simulink model "flight_sim"  (R2024a)
settings: Solver=VariableStepAuto  StartTime=0.0  StopTime=100  RelTol=1e-3
libraries: aerolibatmos2 x1, matrix_library x1, shared6dof x1
settings Model: Creator=zach  LastModifiedBy=zach

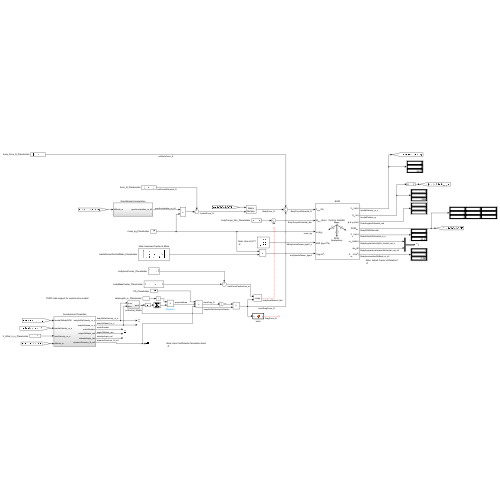
[thumbnail: Simulink's stored preview of the top-level diagram]
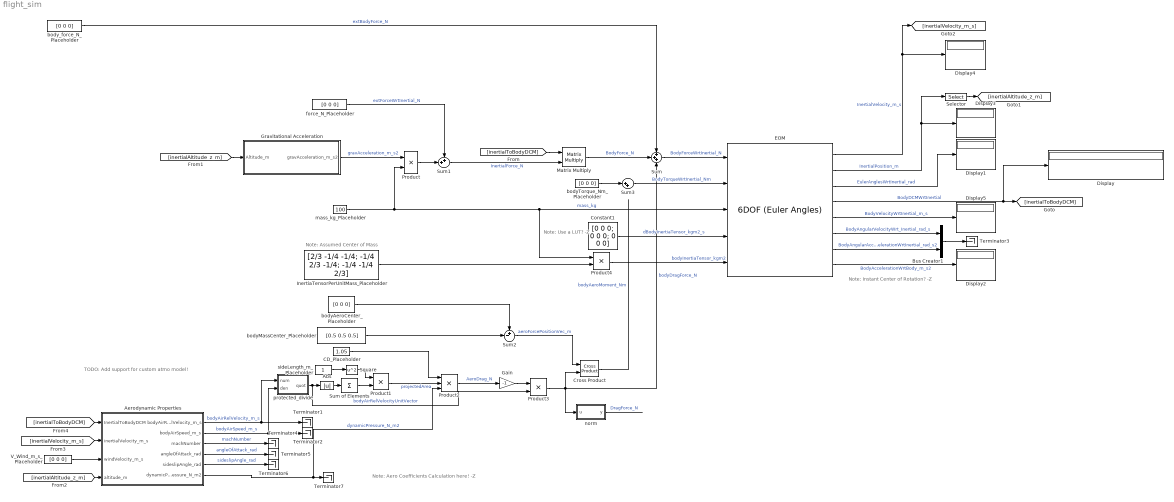
== system flight_sim ==
  note: Note: Assumed Center of Mass
  note: TODO: Add support for custom atmo model!
  note: Note: Aero Coefficients Calculation here!
      |  -Z
  note: Note: Instant Center of Rotation?
      | -Z
  note: Note: Use a LUT?
      | -Z
  Abs : Abs  SaturateOnIntegerOverflow=off
  Aerodynamic Properties : Subsystem
  Bus Creator1 : BusCreator  Inputs=2
  CD_Placeholder : Constant  Value=1.05
  Constant1 : Constant  Value=[0 0 0; 0 0 0; 0 0 0]
  Cross Product : matrix_library/Cross Product
  Display{,1..5} (6 alike) : Display
  EOM : shared6dof/6DOF (Euler Angles)  units=Metric (MKS)  mtype=Custom Variable  rep=Quaternion  xme_0=[0 0 10000]  Vm_0=[0 0 0]  eul_0=[0 0 0]  pm_0=[0 0 0]  mass_0=100  mass_e=0.5  mass_f=100  inertia=eye(3)  inertia_e=eye(3)  inertia_f=2*eye(3)  k_quat=1.0  vre_flag=off  abi_flag=off  aMode=0  xme_statename=''  Vm_statename=''  eul_statename=''  quat_statename=''  pm_statename=''  mass_statename=''
      settings: LibrarySourceBlock=aerolib6dof2/6DOF (Quaternion)
  Gain : Gain  Gain=-1
  Gravitational Acceleration : Subsystem
  InertiaTensorPerUnitMass_Placeholder : Constant  Value=[2/3 -1/4 -1/4; -1/4 2/3 -1/4; -1/4 -1/4 2/3]
  Matrix Multiply : Product  Multiplication=Matrix(*)
  Product{,1,3..4} (4 alike) : Product
  Product2 : Product  Inputs=3
  Selector : Selector  InputPortWidth=3  IndexOptions=Index vector (dialog)  Indices=[3]  OutputSizes=1
  Square : Math  Operator=square
  Sum : Sum  Inputs=+++
  Sum of Elements : Sum  Inputs=+
  Sum1 : Sum  Inputs=++|
  Sum2 : Sum  Inputs=+-|
  Sum3 : Sum  Inputs=|++
  Terminator{1..7} (7 alike) : Terminator
  V_Wind_m_s_Placeholder : Constant  Value=[0 0 0]
  bodyAeroCenter_Placeholder : Constant  Value=[0 0 0]
  bodyMassCenter_Placeholder : Constant  Value=[0.5 0.5 0.5]
  bodyTorque_Nm_Placeholder : Constant  Value=[0 0 0]
  body_force_N_Placeholder : Constant  Value=[0 0 0]
  force_N_Placeholder : Constant  Value=[0 0 0]
  mass_kg_Placeholder : Constant  Value=100
  norm : MATLAB Function  TreatAsAtomicUnit=on
  protected_divide : Subsystem
  sideLength_m_Placeholder : Constant
  wires:
  Sum3/1 -> EOM/2  "BodyTorqueWrtInertial_Nm"
  EOM/3 -> Display1/1  "EulerAnglesWrtInertial_rad"
  EOM/2 -> Selector/1, Display3/1  "InertialPosition_m"
  EOM/1 -> [inertialVelocity_m_s], Display4/1  "InertialVelocity_m_s"
  EOM/4 -> Display/1, [inertialToBodyDCM]  "BodyDCMWrtInertial"
  EOM/5 -> Display5/1  "BodyVelocityWrtInertial_m_s"
  mass_kg_Placeholder/1 -> Product4/1, EOM/3, Product/2  "mass_kg"
  Sum/1 -> EOM/1  "BodyForceWrtInertial_N"
  Constant1/1 -> EOM/4  "dBodyInertiaTensor_kgm2_s"
  Product4/1 -> EOM/5  "bodyInertiaTensor_kgm2"
  Product/1 -> Sum1/2
  EOM/6 -> Bus Creator1/1  "BodyAngularVelocityWrt_Inertial_rad_s"
  EOM/7 -> Bus Creator1/2  "BodyAngularAccelerationWrtInertial_rad_s2"
  Bus Creator1/1 -> Terminator3/1
  EOM/8 -> Display2/1  "BodyAccelerationWrtBody_m_s2"
  body_force_N_Placeholder/1 -> Sum/1  "extBodyForce_N"
  force_N_Placeholder/1 -> Sum1/1  "extForceWrtInertial_N"
  Sum1/1 -> Matrix Multiply/2  "InertialForce_N"
  [inertialToBodyDCM] -> Matrix Multiply/1
  Matrix Multiply/1 -> Sum/2  "BodyForce_N"
  Selector/1 -> [inertialAltitude_z_m]
  [inertialToBodyDCM] -> Aerodynamic Properties/1(InertialToBodyDCM)
  [inertialVelocity_m_s] -> Aerodynamic Properties/2(inertialVelocity_m_s)
  V_Wind_m_s_Placeholder/1 -> Aerodynamic Properties/3(windVelocity_m_s)
  [inertialAltitude_z_m] -> Aerodynamic Properties/4(altitude_m)
  Aerodynamic Properties/2(bodyAirSpeed_m_s) -> Terminator2/1, protected_divide/2(den)  "bodyAirSpeed_m_s"
  Aerodynamic Properties/3(machNumber) -> Terminator4/1  "machNumber"
  Aerodynamic Properties/4(angleOfAttack_rad) -> Terminator5/1  "angleOfAttack_rad"
  Aerodynamic Properties/5(sideslipAngle_rad) -> Terminator6/1  "sideslipAngle_rad"
  Aerodynamic Properties/6(dynamicPressure_N_m2) -> Product2/3, Terminator7/1  "dynamicPressure_N_m2"
  [inertialAltitude_z_m] -> Gravitational Acceleration/1(Altitude_m)
  Gravitational Acceleration/1(gravAcceleration_m_s2) -> Product/1  "gravAcceleration_m_s2"
  sideLength_m_Placeholder/1 -> Square/1
  Aerodynamic Properties/1(bodyAirRelVelocity_m_s) -> Terminator1/1, protected_divide/1(num)  "bodyAirRelVelocity_m_s"
  protected_divide/1(quot) -> Product3/2, Abs/1  "bodyAirRelVelocityUnitVector"
  Abs/1 -> Sum of Elements/1
  Sum of Elements/1 -> Product1/2
  Square/1 -> Product1/1
  Product1/1 -> Product2/2  "projectedArea"
  CD_Placeholder/1 -> Product2/1
  Product2/1 -> Gain/1  "AeroDrag_N"
  Gain/1 -> Product3/1
  Product3/1 -> norm/1(u), Sum/3, Cross Product/2  "bodyDragForce_N"
  InertiaTensorPerUnitMass_Placeholder/1 -> Product4/2
  bodyMassCenter_Placeholder/1 -> Sum2/2
  bodyAeroCenter_Placeholder/1 -> Sum2/1
  Sum2/1 -> Cross Product/1  "aeroForcePositionVec_m"
  Cross Product/1 -> ?  "bodyAeroMoment_Nm"
  bodyTorque_Nm_Placeholder/1 -> Sum3/1
  norm/1(y) -> ?  "DragForce_N"

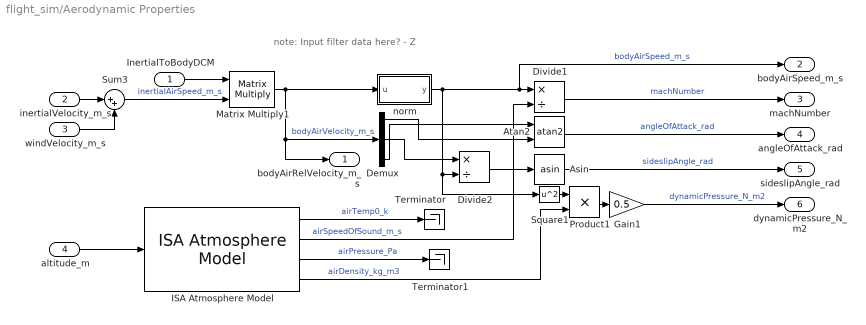
== system flight_sim/Aerodynamic Properties ==
  note: note: Input filter data here?
      |  - Z
  InertialToBodyDCM : Inport
  inertialVelocity_m_s : Inport  Port=2
  windVelocity_m_s : Inport  Port=3
  altitude_m : Inport  Port=4
  Asin : Trigonometry  Operator=asin
  Atan2 : Trigonometry  Operator=atan2
  Demux : Demux  Outputs=3
  Divide1 : Product  Inputs=*/
  Divide2 : Product  Inputs=*/
  Gain1 : Gain  Gain=0.5
  ISA Atmosphere Model : aerolibatmos2/ISA Atmosphere Model  useExtended=off  action=Warning  custom=off  viscosityOut=off  g=9.80665  gamma=1.4  R=287.0531  L=0.0065  h_trop=11000  h_strat=20000  rho0=1.225  P0=101325  T0=288.15  h0=0  S=110.4  Tref=273.15  muref=1.716e-5
  Matrix Multiply1 : Product  Multiplication=Matrix(*)
  Product1 : Product
  Square1 : Math  Operator=square
  Sum3 : Sum  Inputs=|++
  Terminator : Terminator
  Terminator1 : Terminator
  norm : MATLAB Function  TreatAsAtomicUnit=on
  bodyAirRelVelocity_m_s : Outport
  bodyAirSpeed_m_s : Outport  Port=2
  machNumber : Outport  Port=3
  angleOfAttack_rad : Outport  Port=4
  sideslipAngle_rad : Outport  Port=5
  dynamicPressure_N_m2 : Outport  Port=6
  wires:
  Demux/1 -> Atan2/2
  norm/1(y) -> bodyAirSpeed_m_s/1, Divide1/1, Divide2/2, Square1/1  "bodyAirSpeed_m_s"
  ISA Atmosphere Model/2 -> Divide1/2  "airSpeedOfSound_m_s"
  Matrix Multiply1/1 -> bodyAirRelVelocity_m_s/1, Demux/1, norm/1(u)  "bodyAirVelocity_m_s"
  Sum3/1 -> Matrix Multiply1/2  "inertialAirSpeed_m_s"
  Demux/3 -> Atan2/1
  ISA Atmosphere Model/4 -> Product1/2  "airDensity_kg_m3"
  Square1/1 -> Product1/1
  ISA Atmosphere Model/3 -> Terminator1/1  "airPressure_Pa"
  Gain1/1 -> dynamicPressure_N_m2/1  "dynamicPressure_N_m2"
  Demux/2 -> Divide2/1
  Product1/1 -> Gain1/1
  Divide2/1 -> Asin/1
  inertialVelocity_m_s/1 -> Sum3/1
  ISA Atmosphere Model/1 -> Terminator/1  "airTemp0_k"
  Atan2/1 -> angleOfAttack_rad/1  "angleOfAttack_rad"
  InertialToBodyDCM/1 -> Matrix Multiply1/1
  Divide1/1 -> machNumber/1  "machNumber"
  altitude_m/1 -> ISA Atmosphere Model/1
  windVelocity_m_s/1 -> Sum3/2
  Asin/1 -> sideslipAngle_rad/1  "sideslipAngle_rad"

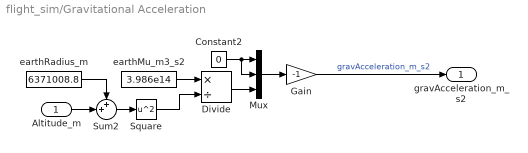
== system flight_sim/Gravitational Acceleration ==
  Altitude_m : Inport
  Constant2 : Constant  Value=0
  Divide : Product  Inputs=*/
  Gain : Gain  Gain=-1
  Mux : Mux  Inputs=3
  Square : Math  Operator=square
  Sum2 : Sum  Inputs=++|
  earthMu_m3_s2 : Constant  Value=3.986e14
  earthRadius_m : Constant  Value=6371008.8
  gravAcceleration_m_s2 : Outport
  wires:
  Square/1 -> Divide/2
  Constant2/1 -> Mux/2, Mux/1
  earthRadius_m/1 -> Sum2/1
  Sum2/1 -> Square/1
  Divide/1 -> Mux/3
  Mux/1 -> Gain/1
  earthMu_m3_s2/1 -> Divide/1
  Gain/1 -> gravAcceleration_m_s2/1  "gravAcceleration_m_s2"
  Altitude_m/1 -> Sum2/2

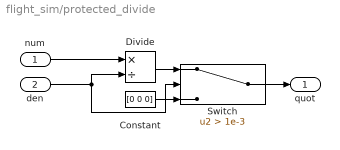
== system flight_sim/protected_divide ==
  num : Inport
  den : Inport  Port=2
  Constant : Constant  Value=[0 0 0]
  Divide : Product  Inputs=*/
  Switch : Switch  Criteria=u2 > Threshold  Threshold=1e-3  SaturateOnIntegerOverflow=off  InputSameDT=off
  quot : Outport
  wires:
  den/1 -> Divide/2, Switch/2
  Constant/1 -> Switch/3
  num/1 -> Divide/1
  Switch/1 -> quot/1
  Divide/1 -> Switch/1

== matlab function flight_sim/Aerodynamic Properties/norm ==
  data: u input; y output
function y = nrm(u)

y = norm(u);

== matlab function flight_sim/norm ==
  data: u input; y output
function y = nrm(u)

y = norm(u);
